simulink model "Narnia_PIL"  (R2023b)
settings: Solver=FixedStepAuto  StartTime=0.0  StopTime=inf  RelTol=1e-3  EnableMultiTasking=on
undefined symbols (not defined in the file or in its folder): A, B, C, DiscIntNeverNeededParam, E
libraries: stm32f4xxblockslib x6, rllib x1, stm32l4xxblockslib x1
settings Model: ExtModeTrigDuration=10  Creator=hdt  LastModifiedBy=hdt
settings OptimizationCC: EnhancedBackFolding=on  PassReuseOutputArgsAs=Individual arguments  ZeroExternalMemoryAtStartup=off  ZeroInternalMemoryAtStartup=off  MaxStackSize=64  OptimizeBlockOrder=speed  DifferentSizesBufferReuse=on  OptimizationCustomize=off  EfficientTunableParamExpr=on
settings DebuggingCC: ParameterTunabilityLossMsg=error
settings HardwareCC: ProdBitPerPointer=32  ProdBitPerSizeT=32  ProdBitPerPtrDiffT=32  ProdLargestAtomicInteger=Long  ProdLargestAtomicFloat=Double  ProdWordSize=32  ProdLongLongMode=on  ProdHWDeviceType=ARM Compatible->ARM Cortex
settings SFSimCC: MATLABDynamicMemAlloc=off  SimTargetLang=C++
settings RTWCC: Description=Embedded Coder  SystemTargetFile=ert.tlc  HardwareBoard=STM32L4xx Based  TemplateMakefile=ert_default_tmf  Toolchain=GNU Tools for ARM Embedded Processors
settings CodeAppCC: ForceParamTrailComments=on  IgnoreCustomStorageClasses=off  OperatorAnnotations=on  SimulinkDataObjDesc=on  SFDataObjDesc=on  InsertBlockDesc=on
settings ERTTargetCC: CodeReplacementLibrary=ARM Cortex-M  ExtModeTransport=3  ExtModeStaticAlloc=on  ExtModeStaticAllocSize=2048  ExtModeMexFile=ext_xcp  ExtModeIntrfLevel=Level2 - Open

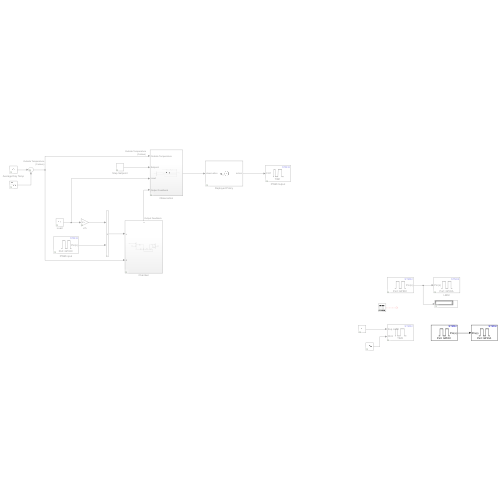
[thumbnail: Simulink's stored preview of the top-level diagram]
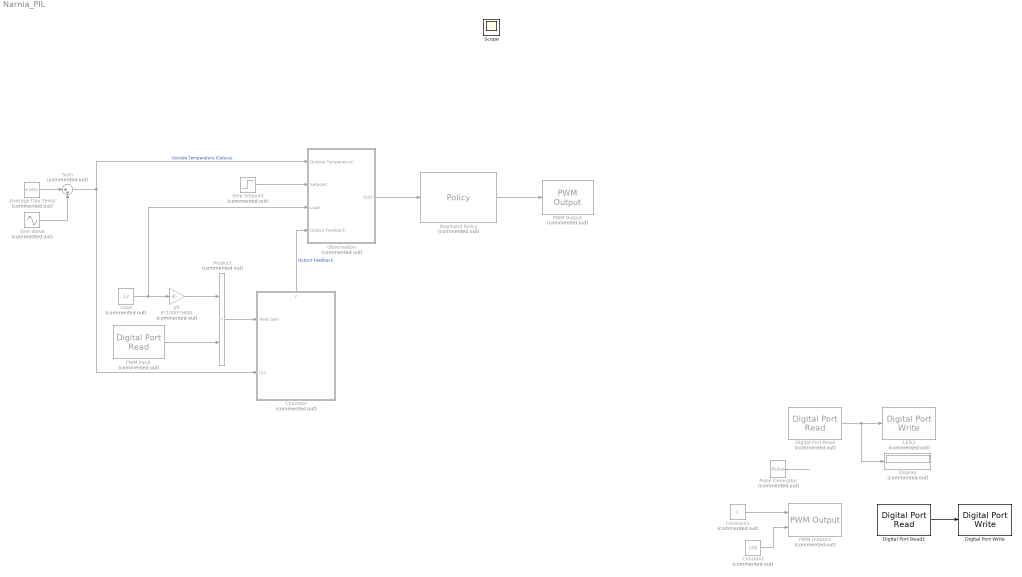
== system Narnia_PIL ==
  Average Day Temp : Constant  Commented=on  Value=8.4801
  Chamber : Subsystem  Commented=on
      settings: PortSchema="{\"entries\":[{\"content\":{\"sides\":[{\"content\":{\"connectorIds\":[\"In1\",\"In2\"]},\"type\":\"ConnectorPlacement.EquallySpacedRectSide\",\"uuid\":\"5c2cfaf1-133f-43fd-8e9c-ee54e397a315\"},{\"content\":{\"side\":\"RIGHT\"},\"type\":\"ConnectorPlacement.EquallySpacedRectSide\",\"uuid\":\"eede310c-e610-4ee9-a639-466ec0e91532\"},{\"content\":{\"connectorIds\":[\"Out1\"],\"side\":\"TOP\"},\"type\":\"ConnectorPlacement.EquallySpacedRectSide\",\"uuid\":\"89ce2564-7231-4560-bf71-cdf8231d8826\"}]},\"type\":\"ConnectorPlacement.EquallySpacedConnector\",\"uuid\":\"cab22b70-b41f-46f9-bd0b-dfcef644d510\"}],\"packageUris\":[\"http://schema.mathworks.com/mf0/Connector/R2020b\"],\"version\":\"1.0\"}"
  Constant : Constant  Commented=on  Value=100
  Constant1 : Constant  Commented=on
  Deployed Policy : rllib/Policy  Commented=on  MATFile=blockAgentData.mat  SimUsingCodegen=off
  Digital Port Read : stm32f4xxblockslib/Digital Port Read  Commented=on  PortName=GPIOC  PinNumber=[1]  ReadOperation=on  IOAsArray=on  SampleTime=-1  EnableSimPort=off
      settings: LibrarySourceBlock=stm32l4xxblockslib/Digital Port Read
  Digital Port Read1 : stm32f4xxblockslib/Digital Port Read  PortName=GPIOC  PinNumber=[13]  ReadOperation=on  IOAsArray=on  SampleTime=-1  EnableSimPort=off
      settings: LibrarySourceBlock=stm32l4xxblockslib/Digital Port Read
  Digital Port Write : stm32f4xxblockslib/Digital Port Write  PortName=GPIOA  PinNumber=[5]  ReadOperation=off  IOAsArray=on  EnableSimPort=off
      settings: LibrarySourceBlock=stm32l4xxblockslib/Digital Port Write
  Display : Display  Commented=on
  J/h : Gain  Commented=on  Gain=4*1000*3600
  LED2 : stm32f4xxblockslib/Digital Port Write  Commented=on  PortName=GPIOA  PinNumber=[5]  ReadOperation=off  IOAsArray=on  EnableSimPort=off
      settings: LibrarySourceBlock=stm32l4xxblockslib/Digital Port Write
  Load : Constant  Commented=on  Value=12
  Observation : Subsystem  Commented=on
  PWM Output : stm32f4xxblockslib/PWM Output  Commented=on  TimerModule=TIM1  DutycycleUnits=Percentage  EnableChannel1=on  EnableChannel2=off  EnableChannel3=off  EnableChannel4=off  EnableCounterInput=off  EnableMainOutputInput=off  EnableFrequencyInput=off  SetRCAfterCE=off  OutputDirection=off  OutputMainOutputEnableStatus=off  SampleTime=0.1  EnableSimPort=off  EnableUpdateEvent=off  EnableCaptureCompare1Event=off  EnableCaptureCompare2Event=off  EnableCaptureCompare3Event=off  EnableCaptureCompare4Event=off  EnableTriggerEvent=off  EnableBreakEvent=off  ProcessorFamily=STM32F4  hoistedMaskSrc=ECSoC/ECSimCodegen/PWM Output
  PWM Output1 : stm32l4xxblockslib/PWM Output  Commented=on  TimerModule=TIM3  DutycycleUnits=Percentage  EnableChannel1=off  EnableChannel2=on  EnableChannel3=off  EnableChannel4=off  EnableChannel5=off  EnableChannel6=off  EnableCounterInput=off  EnableMainOutputInput=off  EnableFrequencyInput=on  SetRCAfterCE=off  OutputDirection=off  OutputMainOutputEnableStatus=off  SampleTime=0.1  EnableSimPort=off  EnableUpdateEvent=off  EnableCaptureCompare1Event=off  EnableCaptureCompare2Event=off  EnableCaptureCompare3Event=off  EnableCaptureCompare4Event=off  EnableTriggerEvent=off  EnableBreakEvent=off  EnableBreakEvent2=off  ProcessorFamily=STM32L4  hoistedMaskSrc=ECSoC/ECSimCodegen/PWM Output
  PWM input : stm32f4xxblockslib/Digital Port Read  Commented=on  PortName=GPIOC  PinNumber=[13]  ReadOperation=on  IOAsArray=on  SampleTime=-1  EnableSimPort=off
  Product : Product  Commented=on
  Pulse Generator : DiscretePulseGenerator  Commented=on
  Sine Wave : Sin  Commented=on  Amplitude=4  Frequency=pi/12  SampleTime=0
  Step Setpoint : Step  Commented=on  Time=60  Before=24  After=28
  Sum : Sum  Commented=on  Inputs=|++
  Scope : Scope
  wires:
  Deployed Policy/1 -> PWM Output/1
  PWM input/1 -> Product/2
  Product/1 -> Chamber/1(Heat Gain)
  Observation/1(Out1) -> Deployed Policy/1
  Sum/1 -> Chamber/2(In2), Observation/1(Outside Temperature)  "Outside Temperature (Celsius)"
  Average Day Temp/1 -> Sum/1
  Sine Wave/1 -> Sum/2
  Step Setpoint/1 -> Observation/2(Setpoint)
  J/h/1 -> Product/1
  Load/1 -> Observation/3(Load), J/h/1
  Chamber/1(y) -> Observation/4(Output Feedback)  "Output Feedback"
  Constant/1 -> PWM Output1/2
  Digital Port Read/1 -> Display/1, LED2/1
  Pulse Generator/1 -> ?
  Constant1/1 -> PWM Output1/1
  Digital Port Read1/1 -> Digital Port Write/1

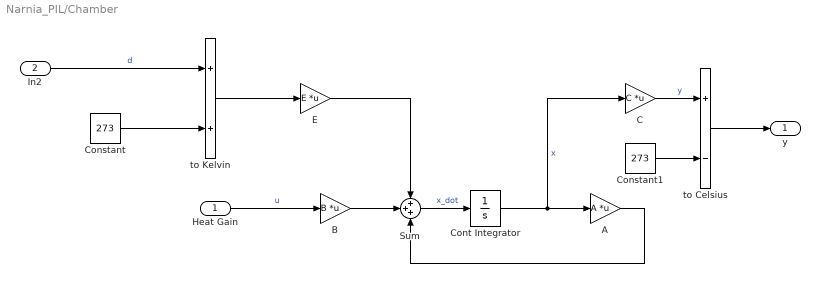
== system Narnia_PIL/Chamber ==
  Heat Gain : Inport  Unit=J/h
  In2 : Inport  Port=2  Unit=Celsius
  A : Gain  Gain=A  Multiplication=Matrix(K*u)
  B : Gain  Gain=B  Multiplication=Matrix(K*u)
  C : Gain  Gain=C  Multiplication=Matrix(K*u)
  Constant : Constant  Value=273
  Constant1 : Constant  Value=273
  Cont Integrator : Integrator  InitialCondition=[19+273;10+273]
  E : Gain  Gain=E  Multiplication=Matrix(K*u)
  Sum : Sum  Inputs=+++
  to Celsius : Sum  Inputs=+-
  to Kelvin : Sum
  y : Outport  Unit=°C
  wires:
  Heat Gain/1 -> B/1  "u"
  B/1 -> Sum/2
  A/1 -> Sum/3
  Sum/1 -> Cont Integrator/1  "x_dot"
  Cont Integrator/1 -> C/1, A/1  "x"
  E/1 -> Sum/1
  In2/1 -> to Kelvin/1  "d"
  C/1 -> to Celsius/1  "y"
  Constant/1 -> to Kelvin/2
  to Kelvin/1 -> E/1
  to Celsius/1 -> y/1
  Constant1/1 -> to Celsius/2

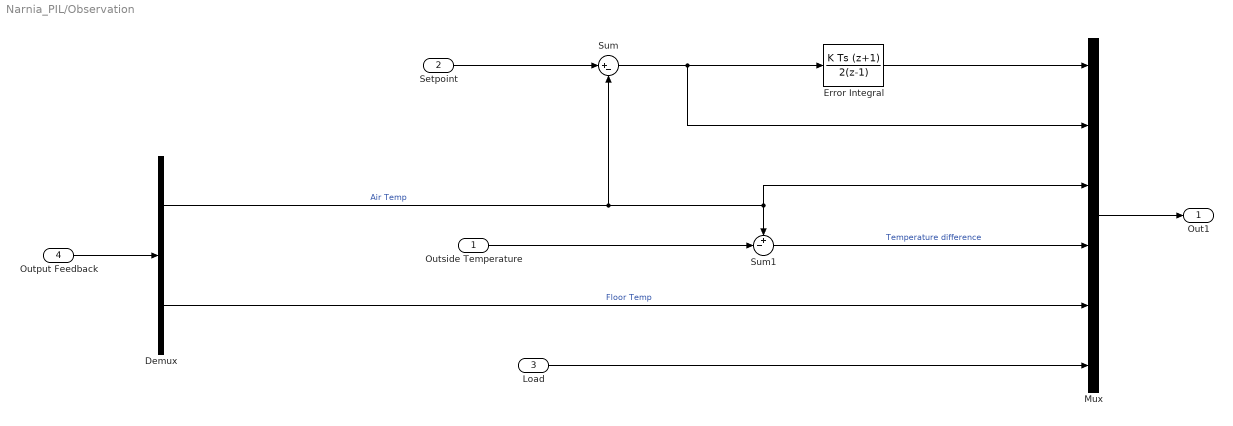
== system Narnia_PIL/Observation ==
  Outside Temperature : Inport  Unit=°C
  Setpoint : Inport  Port=2  Unit=°C
  Load : Inport  Port=3  Unit=A
  Output Feedback : Inport  Port=4  Unit=°C
  Demux : Demux  Outputs=2
  Error Integral : DiscreteIntegrator  IntegratorMethod=Integration: Trapezoidal  SampleTime=-1  ICPrevOutput=DiscIntNeverNeededParam  ICPrevScaledInput=DiscIntNeverNeededParam
  Mux : Mux  Inputs=6
  Sum : Sum  Inputs=|+-
  Sum1 : Sum  Inputs=+-|
  Out1 : Outport
  wires:
  Outside Temperature/1 -> Sum1/2
  Setpoint/1 -> Sum/1
  Error Integral/1 -> Mux/1
  Mux/1 -> Out1/1
  Sum/1 -> Error Integral/1, Mux/2
  Sum1/1 -> Mux/4  "Temperature difference"
  Output Feedback/1 -> Demux/1
  Demux/2 -> Mux/5  "Floor Temp"
  Load/1 -> Mux/6
  Demux/1 -> Sum/2, Sum1/1, Mux/3  "Air Temp"
